simulink library "libCerebusParseInC"  (R2015a)
settings: Solver=FixedStepDiscrete  StartTime=0.0  StopTime=Inf  FixedStep=0.001  RelTol=1e-3
undefined symbols (not defined in the file or in its folder): gcbh, mxpcnbunlink, mxpcrtudprx
libraries: xpciplib x2, xpcnetworkbufferlib x1
settings Model: xpc_rtwmakecfg_data=_xpcetherlib__xpcether8255xlib__xpcetherGbElib__xpcnblib_  Creator=shenoylab  LastModifiedBy=shenoylab
settings SolverCC: EnableConcurrentExecution=on
settings OptimizationCC: BlockReduction=off  OptimizeBlockIOStorage=off  BufferReuse=off  GlobalBufferReuse=off  ExpressionFolding=off  LocalBlockOutputs=off
settings HardwareCC: ProdIntDivRoundTo=Zero  ProdEndianess=LittleEndian  ProdLongLongMode=on  ProdHWDeviceType=Generic->32-bit x86 compatible
settings ModelReferenceCC: ModelReferenceNumInstancesAllowed=Single
settings RTWCC: SystemTargetFile=slrt.tlc  TemplateMakefile=slrt_default_tmf  Description=Simulink Real-Time  RTWCompilerOptimization=on
settings CodeAppCC: MaxIdLength=100  MATLABSourceComments=on
settings SimulinkRealTimeCC: GeneratePreprocessorConditionals=Disable all

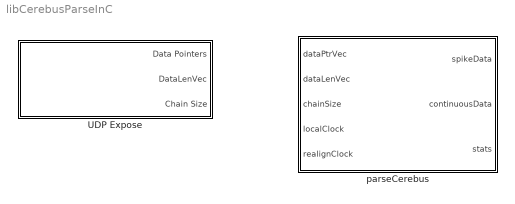
== system libCerebusParseInC ==
  UDP Expose : Subsystem  InitFcn=mxpcrtudprx(1, get_param(gcbh, 'ID'));  mask(rtudpreceive){ID=1, Receive1=0.0.0.0, Receive2=1002, maxPackets=1000, Receive4=0.001, udpID=0}
      mask prompts: ID "Device ID:"; Receive1 "Source IP Address:"; Receive2 "Local (destination) port:"; maxPackets "Max Packets"; Receive4 "Sample time:"; udpID "Internal UDP ID:"
      mask help:
      | Receive data over UDP network on a dedicated network interface.
      |
      | This block receives data on the specified local (destination) port. To receive all data sent to this port, set 'Source IP Address' to 0.0.0.0. To receive data sent to this port from a specific remote source, enter the IP address of that source.
      mask init:
      | Receive1 = ipaddr(Receive1);
      | udpID = ID -1;
      mask Help: eval('xpcdoc(''RT_UDP_RECEIVE'')');
      mask TypeOptions ID: 1 | 2 | 3 | 4 | 5 | 6 | 7 | 8
      mask Display:
      | disp(sprintf('UDP Expose\nId: %d', ID));
      | port_label('output', 1, 'DataPtrVec');
      | port_label('output', 2, 'DataLenVec');
      | port_label('output', 3, 'Chain Size');
  parseCerebus : MATLAB Function  TreatAsAtomicUnit=on

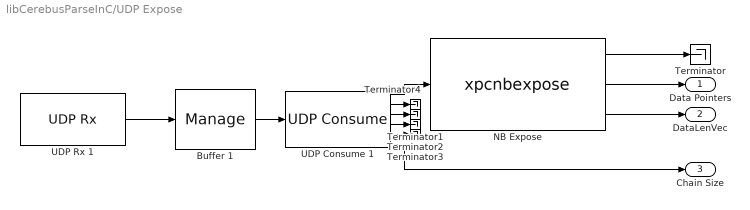
== system libCerebusParseInC/UDP Expose ==
  Buffer 1 : xpcnetworkbufferlib/Manage   ChainSize=maxPackets  BufferSize=0  Threshold=0
  NB Expose : S-Function  InitFcn=mxpcnbunlink(1,0);  FunctionName=xpcnbexpose  Parameters=vectorLength  mask(xpcnbunlink){VectorLength=maxPackets}
      mask prompts: VectorLength "Vector length (-1 inherit):"
      mask help: Unlink a chain into a vector of network buffers.
      mask init:
      | [vectorLength] = mxpcnbunlink(2, VectorLength);
      mask Help: eval('xpcdoc(''NB_Unlink'')');
      mask Display:
      | disp('NB Expose');
      | port_label('output', 1, 'NBVec');
      | port_label('output', 2, 'DataPtrVec');
      | port_label('output', 3, 'DataLenVec');
  Terminator{,1..4} (5 alike) : Terminator
  UDP Consume 1 : xpciplib/UDP Consume   Group=udpID  VectorSize=maxPackets  SampleTime=Receive4
  UDP Rx 1 : xpciplib/UDP Rx   Priority=5  Group=udpID  sip=Any  SourceAddress=Receive1  lup=Specify  LocalPort=Receive2  SampleTime=Receive4
  Data Pointers : Outport
  DataLenVec : Outport  Port=2
  Chain Size : Outport  Port=3
  wires:
  UDP Consume 1/1 -> NB Expose/1
  Buffer 1/1 -> UDP Consume 1/1
  UDP Rx 1/1 -> Buffer 1/1
  UDP Consume 1/6 -> Chain Size/1
  NB Expose/1 -> Terminator/1
  NB Expose/2 -> Data Pointers/1
  NB Expose/3 -> DataLenVec/1
  UDP Consume 1/3 -> Terminator1/1
  UDP Consume 1/4 -> Terminator2/1
  UDP Consume 1/5 -> Terminator3/1
  UDP Consume 1/2 -> Terminator4/1

== matlab function libCerebusParseInC/parseCerebus ==
  data: dataPtrVec input uint32; dataLenVec input uint32; chainSize input size=1; spikeData output Bus: SpikeDataBus size=1; continuousData output Bus: ContinuousDataBus size=1; stats output Bus: CerebusStatisticsBus size=1; localClock input uint32 size=1; realignClock input size=1; CerebusInfo parameter size=1
function [spikeData, continuousData, stats] = parseCerebus(dataPtrVec, dataLenVec, chainSize, localClock, realignClock, CerebusInfo)
%#codegen

% these pointers are coder.opaque, they will be used only via ceval calls
% within CerebusParse
% [pp, pBufferEnd] = CerebusParse.nbExtractPacketData(nb);

% length of a spike cbPKT in the lab (96 bytes for the waveform, 4 bytes for
% the min and max in the waveform, 12 bytes for spike sorting details
% giving a total of 112 bytes

    % for aligning cerebus clock (30 kHz) to local clock (1 kHz) at start of each trial
    persistent pCerebusClockReference;
    persistent pCerebusClockRecent;
    persistent pLocalClockReference;
    if isempty(pCerebusClockReference)
        pCerebusClockReference = uint32(0);
        pLocalClockReference = uint32(0);
        pCerebusClockRecent = uint32(0);
    end 

    cb_time = uint32(0);
    msOffset = single(0);

    % build the SpikeDataBus fields as full-size copies here
    spikeTimeOffsets = zeros([CerebusInfo.MaxSpikesPerTick 1], 'single');
    spikeChannels = zeros([CerebusInfo.MaxSpikesPerTick 1], 'uint8');
    spikeUnits = zeros([CerebusInfo.MaxSpikesPerTick 1], 'uint8');
    spikeWaveforms = zeros([CerebusInfo.WaveformNumSamples CerebusInfo.MaxSpikesPerTick], 'int16');
    
    % build the ContinuousDataBus fields as full-size copies here
    continuousTimeOffsets = zeros([CerebusInfo.MaxChannels 1], 'single');
    continuousSamples = zeros([CerebusInfo.MaxChannels CerebusInfo.MaxContinuousSamplesPerTick], 'int16');
    
    stats = initializeBus_CerebusStatisticsBus();
    stats.nSpikes = uint32(0);
    stats.nContinuousChannels = uint16(0);
    stats.nContinuousSamples = uint32(0);
    stats.nCBPackets = uint32(0);

    for iP = uint32(1):uint32(chainSize)
        if dataPtrVec(iP) == 0 || dataLenVec(iP) == 0
            continue;
        end

        stats.nUDPPackets = stats.nUDPPackets + uint32(1);
        stats.nUDPBytes = stats.nUDPBytes + uint32(dataLenVec(iP));
        
        [pp, pBufferEnd] = CerebusParse.getPointersFromDataPtr(dataPtrVec(iP), dataLenVec(iP));
        stats.nCBPackets = stats.nCBPackets + uint32(1);

        while true
            cb_time = CerebusParse.getTime(pp);
            
            % on the first cbPKT received,
            % reset the clock alignment after the buffer has been flushed of old packets
            % and if starting a new trial.
            if cb_time > 0 && localClock > 10 && (pCerebusClockReference == 0 || realignClock)
                % reset the clock alignment between local (1 kHz) and Cerebus (30 kHz)
                % typically at the end of trials
                pCerebusClockReference = cb_time;
                pLocalClockReference = localClock;
                %coder.ceval('printf', [char('Cerebus align cc %g, lc %g') 10 0], pCerebusClockReference, pLocalClockReference);
            end

            if CerebusParse.isSpikePacket(pp)
                % Received spike packet
                if stats.nSpikes < uint32(CerebusInfo.MaxSpikesPerTick)
                    stats.nSpikes = stats.nSpikes + uint32(1);

                    cb_channel = CerebusParse.getChannel(pp);
                    cb_unit = CerebusParse.getSpikeUnit(pp);

                    if cb_channel >= 1 && cb_channel <= CerebusInfo.MaxChannels
                       msOffset = CerebusParse.computeTimeOffsetMs(cb_time, localClock, ...
                           pLocalClockReference, pCerebusClockReference);

                        % store spike info and waveform
                        spikeTimeOffsets(stats.nSpikes) = msOffset;
                        spikeChannels(stats.nSpikes) = cb_channel;
                        spikeUnits(stats.nSpikes) = cb_unit;
                        
                        % copy spike waveform directly into waveforms matrix
                        spikeWaveforms = CerebusParse.copySpikeWaveformToBufferColumn(pp, spikeWaveforms, stats.nSpikes);
                        
                        % update statistics
                        stats.nSpikesByChannel(cb_channel) = stats.nSpikesByChannel(cb_channel) + uint32(1);
                    end
                end

            elseif CerebusParse.isContinuousPacketForGroup(pp, uint8(CerebusInfo.ContinuousGroupId))
                % receieved continuous data sample for the appropriate group id
                if stats.nContinuousSamples < uint32(CerebusInfo.MaxContinuousSamplesPerTick)
                    stats.nContinuousSamples = stats.nContinuousSamples + uint32(1);

                    msOffset = CerebusParse.computeTimeOffsetMs(cb_time, localClock, ...
                           pLocalClockReference, pCerebusClockReference);

                    continuousTimeOffsets(stats.nContinuousSamples) = msOffset;

                    if stats.nContinuousChannels == uint16(0)
                        % because the number of continuous channels is not known ahead of time,
                        % declare the size of continuousData now that we
                        % have a non-zero channel count
                        stats.nContinuousChannels = uint16(min(CerebusInfo.MaxChannels, CerebusParse.getContinuousNumChannels(pp)));
                    end
                    
                    % copy in the samples
                    continuousSamples = CerebusParse.copyContinuousSamplesToBufferColumn(pp, continuousSamples, stats.nContinuousSamples);
                end
            end

            % jump to the next cbPKT
            if ~CerebusParse.hasNext(pp, pBufferEnd)
                break;
            end
            pp = CerebusParse.getNext(pp);
            stats.nCBPackets = stats.nCBPackets + uint32(1);
        end
    end
    
    % build SpikeDataBus
    spikeData.spikeTimeOffsets = spikeTimeOffsets(1:stats.nSpikes);
    spikeData.spikeChannels = spikeChannels(1:stats.nSpikes);
    spikeData.spikeUnits = spikeUnits(1:stats.nSpikes);
    spikeData.spikeWaveforms = spikeWaveforms(:, 1:stats.nSpikes);

    % build ContinuousDataBus
    continuousData.continuousTimeOffsets = continuousTimeOffsets(1:stats.nContinuousSamples);
    continuousData.continuousData = continuousSamples(1:stats.nContinuousChannels, 1:stats.nContinuousSamples);
    
    if cb_time > uint32(0)
        pCerebusClockRecent = cb_time;
    end
    stats.cerebusClock = pCerebusClockRecent;
    stats.clockOffset = msOffset;

    % store the most recent continuous sample in the stats
    if size(continuousData.continuousData, 2) > 0
        stats.mostRecentContinuousSamples(1:stats.nContinuousChannels) = continuousData.continuousData(1:stats.nContinuousChannels, 1);
    end
    
    stats.cerebusClockRef = pCerebusClockReference;
    stats.localClockRef = pLocalClockReference;
end
